simulink model "PubIfDecisionLM_MDL"  (R2020b)
settings: configuration reference "DspaceConfig" (kept outside this file)
PostLoadFcn:
  | if any(exist('dsrtsu_mdlpostloadfcn', 'file') ~= 0), dsrtsu_mdlpostloadfcn('Execute', bdroot); end
InitFcn:
  | , if any(exist('dsmpb_private', 'file') ~= 0), dsmpb_private('dsmpb_mdlclblib', 'Init', bdroot); end,
undefined symbols (not defined in the file or in its folder): OFM_OBJ_FUSIONTYPE_E, OFM_OBJ_MOVINGSTATE_E, OFM_OBJ_ORIENTATION_E, OFM_OBJ_TYPE_E, P_LM_Cyc, P_LM_EMLHistKapRcdBufSize, P_LM_EMLHistTrajBaseDis, P_LM_EMLHistTrajPNum, P_LM_EMLKapCorrMaxThre, P_LM_EMLMinKapThre, P_LM_EMLPathDisDiffThre, P_LM_EMLQuaFiltPar, P_LM_EMLTurnActKapThre, P_LM_EMLValidQuaThre, P_LM_FntPath1Disgap, P_LM_FntPath1MinDis, P_LM_FntPath1Timegap, P_LM_FntPath2Disgap, P_LM_FntPath2MinDis, P_LM_FntPath2Timegap, P_LM_FntPath3Disgap, P_LM_FntPath3MinDis, P_LM_FntPath3Timegap, P_LM_FusBLParFiltP, P_LM_FusEVDifC2Thre, P_LM_FusEVOPath1AllVSLDisThre, P_LM_FusEVOPath1AllVSLLostNumThre, P_LM_FusEVOPath1AllVSLQuaThre, P_LM_FusEVOPath1OTLFacNLC, P_LM_FusOTLQuaThre, P_LM_FusOTLSW, P_LM_FusParC0Index, P_LM_FusParC1Index, P_LM_FusParC2Index, P_LM_FusParC3Index, P_LM_FusVSLQuaThre, P_LM_FusVSLSW, P_LM_FusVSLValidSteerWheerAngThre, P_LM_FusVSLValidVxvThre, P_LM_LaneWidth, P_LM_OTLBufTPInfoEvaFactor, P_LM_OTLObjNum, P_LM_OTLObjSelectAgeThre, P_LM_OTLObjSelectDxAssessVx, P_LM_OTLObjSelectDxThre, P_LM_OTLObjSelectVxThre, P_LM_OTLObjSelectVyAssessDx, P_LM_OTLObjSelectVyThre, P_LM_OTLTrajPntBaseDis, P_LM_OTLTrajStdThre, P_LM_VSLAvailLineNum, P_LM_VSLBLSDiffThre, P_LM_VSLBLSDisRatio, P_LM_VSLFusBLParFiltP_C1, P_LM_VSLFusBLParFiltP_C2, P_LM_VSLFusBLParFiltP_C3, P_LM_VSLFusBLParFiltP_Quality, P_LM_VSLHistTrajBaseDis, P_LM_VSLHistTrajPNum, P_LM_VSLLCC0diff ... (+18)
libraries: simulink x145, LM_LIB x43
(part 5 of 24)

== system PubIfDecisionLM_MDL/Subsystem2/LM_OTL/LM_OTL_MovObjTrajRecord3/LM_OTL_BufTPCC ==
  LM_OTLBufTPVectBusK1 : Inport
  LM_VCAN_ESP : Inport  Port=2
  LM_ComBus : Inport  Port=3
  Bus Creator : BusCreator  Inputs=12
  Bus Selector : BusSelector  OutputSignals=LM_OTLBufL1DxVect,LM_OTLBufL1DyVect,LM_OTLBufL2DxVect,LM_OTLBufL2DyVect,LM_OTLBufE1DxVect,LM_OTLBufE1DyVect,LM_OTLBufE2DxVect,LM_OTLBufE2DyVect,LM_OTLBufR1DxVect,LM_OTLBufR1DyVect,LM_OTLBufR2DxVect,LM_OTLBufR2DyVect
  Bus Selector2 : BusSelector  OutputSignals=signal7.LM_ComEVOffsetX,signal7.LM_ComEVOffsetY,signal7.LM_ComEVOffsetAng
  Bus Selector5 : BusSelector  OutputSignals=VehStandstill
  Subsystem : Subsystem
  LM_OTLBufTPVectAdjuBus : Outport
  wires:
  LM_OTLBufTPVectBusK1/1 -> Bus Selector/1
  Subsystem/1(LM_OTLBufL1DxVectK1Adju) -> Bus Creator/1  "LM_OTLBufL1DxVectK1Adju"
  Bus Selector/11 -> Subsystem/15(LM_OTLBufR2DxVectK1)  "<LM_OTLBufR2DxVect>"
  Bus Selector/4 -> Subsystem/8(LM_OTLBufL2DyVectK1)  "<LM_OTLBufL2DyVect>"
  Bus Selector/5 -> Subsystem/9(LM_OTLBufE1DxVectK1)  "<LM_OTLBufE1DxVect>"
  Subsystem/5(LM_OTLBufE1DxVectK1Adju) -> Bus Creator/5  "LM_OTLBufE1DxVectK1Adju"
  Bus Selector/10 -> Subsystem/14(LM_OTLBufR1DyVectK1)  "<LM_OTLBufR1DyVect>"
  Bus Selector/8 -> Subsystem/12(LM_OTLBufE2DyVectK1)  "<LM_OTLBufE2DyVect>"
  Bus Selector/9 -> Subsystem/13(LM_OTLBufR1DxVectK1)  "<LM_OTLBufR1DxVect>"
  Bus Selector/7 -> Subsystem/11(LM_OTLBufE2DxVectK1)  "<LM_OTLBufE2DxVect>"
  Bus Selector/6 -> Subsystem/10(LM_OTLBufE1DyVectK1)  "<LM_OTLBufE1DyVect>"
  LM_VCAN_ESP/1 -> Bus Selector5/1
  Bus Selector/3 -> Subsystem/7(LM_OTLBufL2DxVectK1)  "<LM_OTLBufL2DxVect>"
  Subsystem/4(LM_OTLBufL2DyVectK1Adju) -> Bus Creator/4  "LM_OTLBufL2DyVectK1Adju"
  Bus Selector/2 -> Subsystem/6(LM_OTLBufL1DyVectK1)  "<LM_OTLBufL1DyVect>"
  Bus Selector/1 -> Subsystem/5(LM_OTLBufL1DxVectK1)  "<LM_OTLBufL1DxVect>"
  Subsystem/12(LM_OTLBufR2DyVectK1Adju) -> Bus Creator/12  "LM_OTLBufR2DyVectK1Adju"
  Subsystem/7(LM_OTLBufE2DxVectK1Adju) -> Bus Creator/7  "LM_OTLBufE2DxVectK1Adju"
  Subsystem/8(LM_OTLBufE2DyVectK1Adju) -> Bus Creator/8  "LM_OTLBufE2DyVectK1Adju"
  Subsystem/10(LM_OTLBufR1DyVectK1Adju) -> Bus Creator/10  "LM_OTLBufR1DyVectK1Adju"
  Bus Creator/1 -> LM_OTLBufTPVectAdjuBus/1  "LM_OTLBufTPVectAdjuBus"
  Bus Selector/12 -> Subsystem/16(LM_OTLBufR2DyVectK1)  "<LM_OTLBufR2DyVect>"
  Subsystem/9(LM_OTLBufR1DxVectK1Adju) -> Bus Creator/9  "LM_OTLBufR1DxVectK1Adju"
  Subsystem/6(LM_OTLBufE1DyVectK1Adju) -> Bus Creator/6  "LM_OTLBufE1DyVectK1Adju"
  Subsystem/11(LM_OTLBufR2DxVectK1Adju) -> Bus Creator/11  "LM_OTLBufR2DxVectK1Adju"
  Subsystem/2(LM_OTLBufL1DyVectK1Adju) -> Bus Creator/2  "LM_OTLBufL1DyVectK1Adju"
  Subsystem/3(LM_OTLBufL2DxVectK1Adju) -> Bus Creator/3  "LM_OTLBufL2DxVectK1Adju"
  Bus Selector2/1 -> Subsystem/2(LM_OTLOffsetX)  "<LM_ComEVOffsetX>"
  Bus Selector2/2 -> Subsystem/3(LM_OTLOffsetY)  "<LM_ComEVOffsetY>"
  Bus Selector2/3 -> Subsystem/4(LM_OTLOffsetAng)  "<LM_ComEVOffsetAng>"
  LM_ComBus/1 -> Bus Selector2/1
  Bus Selector5/1 -> Subsystem/1(VehStandstill)  "<VehStandstill>"

== system PubIfDecisionLM_MDL/Subsystem2/LM_OTL/LM_OTL_MovObjTrajRecord3/LM_OTL_MovObjSelc ==
  vxvRefMs : Inport
  OFM_OBJS : Inport  Port=2  OutDataTypeStr=Bus: OFM_OBJ_BUS
  Bus Creator : BusCreator  Inputs=6
  Bus Selector : BusSelector  OutputSignals=Object_DX,Object_DY
  Bus Selector1 : BusSelector  OutputSignals=Object_ID,Object_Type,Object_MovingState,Object_VX,Object_Orientation,Object_Fus_Type,Object_ExistProb,Object_VY,Object_DX,Object_Age
  Constant1 : Constant  Value=P_LM_OTLObjNum  OutDataTypeStr=uint8
  Data Type Conversion{,1..5} (6 alike) : DataTypeConversion  OutDataTypeStr=uint8
  LM_OTL_MovObjInterestedSelc : Subsystem
  Subsystem3 : Subsystem
  LM_OTLInterestObjIndexBus : Outport
  wires:
  vxvRefMs/1 -> Subsystem3/1(vxvRefMs)  "vxvRefMs"
  OFM_OBJS/1 -> Bus Selector/1, Bus Selector1/1
  Bus Selector1/10 -> Subsystem3/11(<Object_Age>)  "<Object_Age>"
  Bus Selector1/9 -> Subsystem3/10(<Object_DX>)  "<Object_DX>"
  Bus Selector1/8 -> Subsystem3/9(<Object_VY>)  "<Object_VY>"
  Bus Selector1/7 -> Subsystem3/8(<Object_ExistProb>)  "<Object_ExistProb>"
  Bus Selector1/6 -> Subsystem3/7(<Object_Fus_Type>)  "<Object_Fus_Type>"
  Bus Selector1/5 -> Subsystem3/6(<Object_Orientation>)  "<Object_Orientation>"
  Bus Selector1/4 -> Subsystem3/5(<Object_VX>)  "<Object_VX>"
  Bus Selector1/3 -> Subsystem3/4(<Object_MovingState>)  "<Object_MovingState>"
  Bus Selector1/2 -> Subsystem3/3(<Object_Type>)  "<Object_Type>"
  Bus Selector1/1 -> Subsystem3/2(<Object_ID>)  "<Object_ID>"
  Bus Selector/2 -> LM_OTL_MovObjInterestedSelc/4(Object_DY)  "<Object_DY>"
  Bus Selector/1 -> LM_OTL_MovObjInterestedSelc/3(Object_DX)  "<Object_DX>"
  Bus Creator/1 -> LM_OTLInterestObjIndexBus/1  "LM_OTLObjIndex"
  LM_OTL_MovObjInterestedSelc/6(LM_OTLRigObj2Index) -> Data Type Conversion5/1
  LM_OTL_MovObjInterestedSelc/5(LM_OTLRigObj1Index) -> Data Type Conversion4/1
  LM_OTL_MovObjInterestedSelc/4(LM_OTLHostObj2Index) -> Data Type Conversion3/1
  LM_OTL_MovObjInterestedSelc/3(LM_OTLHostObj1Index) -> Data Type Conversion2/1
  LM_OTL_MovObjInterestedSelc/2(LM_OTLLeObj2Index) -> Data Type Conversion1/1
  LM_OTL_MovObjInterestedSelc/1(LM_OTLLeObj1Index) -> Data Type Conversion/1
  Subsystem3/1(LM_OTL_MovObjValid) -> LM_OTL_MovObjInterestedSelc/1(LM_OTL_MovObjValid)  "LM_OTL_MovObjValid"
  Constant1/1 -> LM_OTL_MovObjInterestedSelc/2(P_LM_ObjNum)
  Data Type Conversion/1 -> Bus Creator/1  "LM_OTLCurLeLaObj1Index"
  Data Type Conversion1/1 -> Bus Creator/2  "LM_OTLCurLeLaObj2Index"
  Data Type Conversion2/1 -> Bus Creator/3  "LM_OTLCurEgoLaObj1Index"
  Data Type Conversion4/1 -> Bus Creator/5  "LM_OTLCurRigLaObj1Index"
  Data Type Conversion5/1 -> Bus Creator/6  "LM_OTLCurRigLaObj2Index"
  Data Type Conversion3/1 -> Bus Creator/4  "LM_OTLCurEgoLaObj2Index"

== system PubIfDecisionLM_MDL/Subsystem2/LM_OTL/LM_OTL_MovObjTrajRecord3/LM_OTL_ObjAlreadyRcdedJudge ==
  note: 判断当前周期感兴趣目标是否已经存储
  Object_ID : Inport  BusOutputAsStruct=on
  LM_OTLBufTPInfoBusK1 : Inport  Port=2
  LM_OTLInterestObjIndexBus : Inport  Port=3
  Bus Creator : BusCreator  Inputs=6
  Bus Creator1 : BusCreator  Inputs=6
  Bus Selector : BusSelector  OutputSignals=LM_OTLCurLeLaObj1Index,LM_OTLCurLeLaObj2Index,LM_OTLCurEgoLaObj1Index,LM_OTLCurEgoLaObj2Index,LM_OTLCurRigLaObj1Index,LM_OTLCurRigLaObj2Index
  Bus Selector1 : BusSelector  OutputSignals=LM_OTLCurLeLaObj1ID,LM_OTLCurLeLaObj2ID
  Bus Selector2 : BusSelector  OutputSignals=LM_OTLBufObjIDInfo.LM_OTLBufL1ObjID,LM_OTLBufObjIDInfo.LM_OTLBufL2ObjID
  Bus Selector3 : BusSelector  OutputSignals=LM_OTLCurEgoLaObj1ID,LM_OTLCurEgoLaObj2ID
  Bus Selector4 : BusSelector  OutputSignals=LM_OTLCurRigLaObj1ID,LM_OTLCurRigLaObj2ID
  Bus Selector5 : BusSelector  OutputSignals=LM_OTLBufObjIDInfo.LM_OTLBufE1ObjID,LM_OTLBufObjIDInfo.LM_OTLBufE2ObjID
  Bus Selector6 : BusSelector  OutputSignals=LM_OTLBufObjIDInfo.LM_OTLBufR1ObjID,LM_OTLBufObjIDInfo.LM_OTLBufR2ObjID
  LM_OTL_CurObjIDCalc : Subsystem
  LM_OTL_EglLaneRcdJudge : Subsystem
  LM_OTL_LeLaneRcdJudge : Subsystem
  LM_OTL_RigLaneRcdJudge : Subsystem
  LM_OTLCurObjIDBus : Outport
  LM_OTLObjRcdedFlg_Bus : Outport  Port=2
  wires:
  LM_OTLInterestObjIndexBus/1 -> Bus Selector/1
  LM_OTL_LeLaneRcdJudge/1(LM_OTLCurLeLaObj1RcdedFlg) -> Bus Creator/1
  LM_OTL_LeLaneRcdJudge/2(LM_OTLCurLeLaObj2RcdedFlg) -> Bus Creator/2
  LM_OTL_EglLaneRcdJudge/1(LM_OTLCurEgoLaObj1RcdedFlg) -> Bus Creator/3
  LM_OTL_EglLaneRcdJudge/2(LM_OTLCurEgoLaObj2RcdedFlg) -> Bus Creator/4
  LM_OTL_RigLaneRcdJudge/1(LM_OTLCurRigLaObj1RcdedFlg) -> Bus Creator/5
  LM_OTL_RigLaneRcdJudge/2(LM_OTLCurRigLaObj2RcdedFlg) -> Bus Creator/6
  Bus Creator/1 -> LM_OTLObjRcdedFlg_Bus/1  "LM_OTLObjRcdedFlg_Bus"
  Object_ID/1 -> LM_OTL_CurObjIDCalc/1(Object_ID)
  Bus Selector/1 -> LM_OTL_CurObjIDCalc/2(LM_OTLCurLeLaObj1Index)  "<LM_OTLCurLeLaObj1Index>"
  Bus Selector/2 -> LM_OTL_CurObjIDCalc/3(LM_OTLCurLeLaObj2Index)  "<LM_OTLCurLeLaObj2Index>"
  Bus Selector/3 -> LM_OTL_CurObjIDCalc/4(LM_OTLCurEgoLaObj1Index)  "<LM_OTLCurEgoLaObj1Index>"
  Bus Selector/4 -> LM_OTL_CurObjIDCalc/5(LM_OTLCurEgoLaObj2Index)  "<LM_OTLCurEgoLaObj2Index>"
  Bus Selector/5 -> LM_OTL_CurObjIDCalc/6(LM_OTLCurRigLaObj1Index)  "<LM_OTLCurRigLaObj1Index>"
  Bus Selector/6 -> LM_OTL_CurObjIDCalc/7(LM_OTLCurRigLaObj2Index)  "<LM_OTLCurRigLaObj2Index>"
  LM_OTL_CurObjIDCalc/1(LM_OTLCurLeLaObj1ID) -> Bus Creator1/1
  LM_OTL_CurObjIDCalc/2(LM_OTLCurLeLaObj2ID) -> Bus Creator1/2
  LM_OTL_CurObjIDCalc/3(LM_OTLCurEgoLaObj1ID) -> Bus Creator1/3
  LM_OTL_CurObjIDCalc/4(LM_OTLCurEgoLaObj2ID) -> Bus Creator1/4
  LM_OTL_CurObjIDCalc/5(LM_OTLCurRigLaObj1ID) -> Bus Creator1/5
  LM_OTL_CurObjIDCalc/6(LM_OTLCurRigLaObj2ID) -> Bus Creator1/6
  Bus Selector1/1 -> LM_OTL_LeLaneRcdJudge/1(LM_OTLCurLeLa1ObjID)  "<LM_OTLCurLeLaObj1ID>"
  Bus Selector1/2 -> LM_OTL_LeLaneRcdJudge/2(LM_OTLCurLeLa2ObjID)  "<LM_OTLCurLeLaObj2ID>"
  Bus Creator1/1 -> LM_OTLCurObjIDBus/1, Bus Selector4/1, Bus Selector3/1, Bus Selector1/1
  LM_OTLBufTPInfoBusK1/1 -> Bus Selector6/1, Bus Selector5/1, Bus Selector2/1
  Bus Selector2/1 -> LM_OTL_LeLaneRcdJudge/3(LM_OTLBufL1ObjIDK1)  "<LM_OTLBufL1ObjID>"
  Bus Selector2/2 -> LM_OTL_LeLaneRcdJudge/4(LM_OTLBufL2ObjIDK1)  "<LM_OTLBufL2ObjID>"
  Bus Selector3/1 -> LM_OTL_EglLaneRcdJudge/1(LM_OTLCurEgoLa1ObjID)  "<LM_OTLCurEgoLaObj1ID>"
  Bus Selector3/2 -> LM_OTL_EglLaneRcdJudge/2(LM_OTLCurEgoLa2ObjID)  "<LM_OTLCurEgoLaObj2ID>"
  Bus Selector4/1 -> LM_OTL_RigLaneRcdJudge/1(LM_OTLCurRigLa1ObjID)  "<LM_OTLCurRigLaObj1ID>"
  Bus Selector4/2 -> LM_OTL_RigLaneRcdJudge/2(LM_OTLCurRigLa2ObjID)  "<LM_OTLCurRigLaObj2ID>"
  Bus Selector5/1 -> LM_OTL_EglLaneRcdJudge/3(LM_OTLBufE1ObjIDK1)  "<LM_OTLBufE1ObjID>"
  Bus Selector5/2 -> LM_OTL_EglLaneRcdJudge/4(LM_OTLBufE2ObjIDK1)  "<LM_OTLBufE2ObjID>"
  Bus Selector6/1 -> LM_OTL_RigLaneRcdJudge/3(LM_OTLBufR1ObjIDK1)  "<LM_OTLBufR1ObjID>"
  Bus Selector6/2 -> LM_OTL_RigLaneRcdJudge/4(LM_OTLBufR2ObjIDK1)  "<LM_OTLBufR2ObjID>"

== system PubIfDecisionLM_MDL/Subsystem2/LM_OTL/LM_OTL_MovObjTrajRecord3/LM_OTL_ObjRcdFlgJudge ==
  LM_OTLObjRcdedFlg_Bus : Inport
  Object_Dx : Inport  Port=2
  Object_Dy : Inport  Port=3
  LM_OTLInterestObjIndexBus : Inport  Port=4
  LM_OTLBufTPVectAdjuBus : Inport  Port=5
  LM_OTLBufTPInfoBusK1 : Inport  Port=6
  Bus Creator : BusCreator  Inputs=12
  Bus Creator1 : BusCreator  Inputs=6
  Bus Creator2 : BusCreator  Inputs=6
  Bus Selector : BusSelector  OutputSignals=LM_OTLCurLeLaObj1RcdedFlg,LM_OTLCurLeLaObj2RcdedFlg
  Bus Selector1 : BusSelector  OutputSignals=LM_OTLCurEgoLaObj1RcdedFlg,LM_OTLCurEgoLaObj2RcdedFlg
  Bus Selector10 : BusSelector  OutputSignals=LM_OTLBufLe1ObjDxK1,LM_OTLBufLe2ObjDxK1
  Bus Selector11 : BusSelector  OutputSignals=LM_OTLBufEgo1ObjDxK1,LM_OTLBufEgo2ObjDxK1
  Bus Selector12 : BusSelector  OutputSignals=LM_OTLBufRig1ObjDxK1,LM_OTLBufRig2ObjDxK1
  Bus Selector13 : BusSelector  OutputSignals=LM_OTLBufL1DxVectK1Adju,LM_OTLBufL2DxVectK1Adju,LM_OTLBufE1DxVectK1Adju,LM_OTLBufE2DxVectK1Adju,LM_OTLBufR1DxVectK1Adju,LM_OTLBufR2DxVectK1Adju
  Bus Selector14 : BusSelector  OutputSignals=LM_OTLBufEPPosInfo.LM_OTLBufL1EPPos,LM_OTLBufEPPosInfo.LM_OTLBufL2EPPos,LM_OTLBufEPPosInfo.LM_OTLBufE1EPPos,LM_OTLBufEPPosInfo.LM_OTLBufE2EPPos,LM_OTLBufEPPosInfo.LM_OTLBufR1EPPos,LM_OTLBufEPPosInfo.LM_OTLBufR2EPPos
  Bus Selector2 : BusSelector  OutputSignals=LM_OTLCurLeLaObj1Index,LM_OTLCurLeLaObj2Index,LM_OTLCurEgoLaObj1Index,LM_OTLCurEgoLaObj2Index,LM_OTLCurRigLaObj1Index,LM_OTLCurRigLaObj2Index
  Bus Selector3 : BusSelector  OutputSignals=LM_OTLCurRigLaObj1RcdedFlg,LM_OTLCurRigLaObj2RcdedFlg
  Bus Selector4 : BusSelector  OutputSignals=LM_OTLCurLeLaObj1Index,LM_OTLCurLeLaObj2Index
  Bus Selector5 : BusSelector  OutputSignals=LM_OTLCurEgoLaObj1Index,LM_OTLCurEgoLaObj2Index
  Bus Selector6 : BusSelector  OutputSignals=LM_OTLCurRigLaObj1Index,LM_OTLCurRigLaObj2Index
  Bus Selector7 : BusSelector  OutputSignals=LM_OTLCurLeLaObj1Dx,LM_OTLCurLeLaObj2Dx
  Bus Selector8 : BusSelector  OutputSignals=LM_OTLCurEgoLaObj1Dx,LM_OTLCurEgoLaObj2Dx
  Bus Selector9 : BusSelector  OutputSignals=LM_OTLCurRigLaObj1Dx,LM_OTLCurRigLaObj2Dx
  LM_OTL_BufObjEndDxCalc : Subsystem
  LM_OTL_CurObjDxCalc : Subsystem
  LM_OTL_EgoLaObjRcdFlgJudge : Subsystem
  LM_OTL_LeLaObjRcdFlgJudge : Subsystem
  LM_OTL_RigLaObjRcdFlgJudge : Subsystem
  LM_OTLCurObjRcdFlgBus : Outport
  LM_OTLCurObjPositonBus : Outport  Port=2
  wires:
  Bus Selector14/6 -> LM_OTL_BufObjEndDxCalc/12(LM_OTLBufRig2ObjPEndIndexK1)  "<LM_OTLBufR2EPPos>"
  Bus Selector14/5 -> LM_OTL_BufObjEndDxCalc/11(LM_OTLBufRig1ObjPEndIndexK1)  "<LM_OTLBufR1EPPos>"
  Bus Selector14/4 -> LM_OTL_BufObjEndDxCalc/10(LM_OTLBufEgo2ObjPEndIndexK1)  "<LM_OTLBufE2EPPos>"
  Bus Selector14/3 -> LM_OTL_BufObjEndDxCalc/9(LM_OTLBufEgo1ObjPEndIndexK1)  "<LM_OTLBufE1EPPos>"
  Bus Selector14/2 -> LM_OTL_BufObjEndDxCalc/8(LM_OTLBufLe2ObjPEndIndexK1)  "<LM_OTLBufL2EPPos>"
  Bus Selector14/1 -> LM_OTL_BufObjEndDxCalc/7(LM_OTLBufLe1ObjPEndIndexK1)  "<LM_OTLBufL1EPPos>"
  Bus Selector13/6 -> LM_OTL_BufObjEndDxCalc/6(LM_OTLBufRig2ObjDxVectK1)  "<LM_OTLBufR2DxVectK1Adju>"
  Bus Selector13/5 -> LM_OTL_BufObjEndDxCalc/5(LM_OTLBufRig1ObjDxVectK1)  "<LM_OTLBufR1DxVectK1Adju>"
  Bus Selector13/4 -> LM_OTL_BufObjEndDxCalc/4(LM_OTLBufEgo2ObjDxVectK1)  "<LM_OTLBufE2DxVectK1Adju>"
  Bus Selector13/3 -> LM_OTL_BufObjEndDxCalc/3(LM_OTLBufEgo1ObjDxVectK1)  "<LM_OTLBufE1DxVectK1Adju>"
  Bus Selector13/2 -> LM_OTL_BufObjEndDxCalc/2(LM_OTLBufLe2ObjDxVectK1)  "<LM_OTLBufL2DxVectK1Adju>"
  Bus Selector13/1 -> LM_OTL_BufObjEndDxCalc/1(LM_OTLBufLe1ObjDxVectK1)  "<LM_OTLBufL1DxVectK1Adju>"
  LM_OTLBufTPInfoBusK1/1 -> Bus Selector14/1
  LM_OTLBufTPVectAdjuBus/1 -> Bus Selector13/1
  LM_OTLObjRcdedFlg_Bus/1 -> Bus Selector/1, Bus Selector3/1, Bus Selector1/1
  Bus Selector/1 -> LM_OTL_LeLaObjRcdFlgJudge/1(LM_OTLCurLeLaObj1RcdedFlg)  "<LM_OTLCurLeLaObj1RcdedFlg>"
  Bus Selector/2 -> LM_OTL_LeLaObjRcdFlgJudge/2(LM_OTLCurLeLaObj2RcdedFlg)  "<LM_OTLCurLeLaObj2RcdedFlg>"
  LM_OTLInterestObjIndexBus/1 -> [LM_OTLInterestObjIndexBus], Bus Selector2/1
  Bus Selector2/1 -> LM_OTL_CurObjDxCalc/3(LM_OTLCurLeLaObj1Index)  "<LM_OTLCurLeLaObj1Index>"
  Bus Selector2/2 -> LM_OTL_CurObjDxCalc/4(LM_OTLCurLeLaObj2Index)  "<LM_OTLCurLeLaObj2Index>"
  Bus Selector2/3 -> LM_OTL_CurObjDxCalc/5(LM_OTLCurEgoLaObj1Index)  "<LM_OTLCurEgoLaObj1Index>"
  Bus Selector2/4 -> LM_OTL_CurObjDxCalc/6(LM_OTLCurEgoLaObj2Index)  "<LM_OTLCurEgoLaObj2Index>"
  Bus Selector2/5 -> LM_OTL_CurObjDxCalc/7(LM_OTLCurRigLaObj1Index)  "<LM_OTLCurRigLaObj1Index>"
  Bus Selector2/6 -> LM_OTL_CurObjDxCalc/8(LM_OTLCurRigLaObj2Index)  "<LM_OTLCurRigLaObj2Index>"
  Bus Creator/1 -> LM_OTLCurObjPositonBus/1, Bus Selector7/1, Bus Selector8/1, Bus Selector9/1  "LM_OTLCurObjDxBus"
  Bus Selector1/1 -> LM_OTL_EgoLaObjRcdFlgJudge/1(LM_OTLCurEgoLaObj1RcdedFlg)  "<LM_OTLCurEgoLaObj1RcdedFlg>"
  Bus Selector1/2 -> LM_OTL_EgoLaObjRcdFlgJudge/2(LM_OTLCurEgoLaObj2RcdedFlg)  "<LM_OTLCurEgoLaObj2RcdedFlg>"
  Bus Selector3/1 -> LM_OTL_RigLaObjRcdFlgJudge/7(LM_OTLCurRigLaObj1RcdedFlg)  "<LM_OTLCurRigLaObj1RcdedFlg>"
  Bus Selector3/2 -> LM_OTL_RigLaObjRcdFlgJudge/8(LM_OTLCurRigLaObj2RcdedFlg)  "<LM_OTLCurRigLaObj2RcdedFlg>"
  Object_Dx/1 -> LM_OTL_CurObjDxCalc/1(Object_Dx)
  Bus Selector4/2 -> LM_OTL_LeLaObjRcdFlgJudge/4(LM_OTLCurLeLaObj2Index)  "<LM_OTLCurLeLaObj2Index>"
  Bus Selector4/1 -> LM_OTL_LeLaObjRcdFlgJudge/3(LM_OTLCurLeLaObj1Index)  "<LM_OTLCurLeLaObj1Index>"
  [LM_OTLInterestObjIndexBus] -> Bus Selector5/1, Bus Selector6/1, Bus Selector4/1
  Bus Selector5/1 -> LM_OTL_EgoLaObjRcdFlgJudge/3(LM_OTLCurEgoLaObj1Index)  "<LM_OTLCurEgoLaObj1Index>"
  Bus Selector5/2 -> LM_OTL_EgoLaObjRcdFlgJudge/4(LM_OTLCurEgoLaObj2Index)  "<LM_OTLCurEgoLaObj2Index>"
  Bus Selector6/1 -> LM_OTL_RigLaObjRcdFlgJudge/1(LM_OTLCurRigLaObj1Index)  "<LM_OTLCurRigLaObj1Index>"
  Bus Selector6/2 -> LM_OTL_RigLaObjRcdFlgJudge/2(LM_OTLCurRigLaObj2Index)  "<LM_OTLCurRigLaObj2Index>"
  Bus Selector7/1 -> LM_OTL_LeLaObjRcdFlgJudge/5(LM_OTLCurLeLaObj1Dx)  "<LM_OTLCurLeLaObj1Dx>"
  Bus Selector7/2 -> LM_OTL_LeLaObjRcdFlgJudge/6(LM_OTLCurLeLaObj2Dx)  "<LM_OTLCurLeLaObj2Dx>"
  Bus Selector8/1 -> LM_OTL_EgoLaObjRcdFlgJudge/5(LM_OTLCurEgoLaObj1Dx)  "<LM_OTLCurEgoLaObj1Dx>"
  Bus Selector8/2 -> LM_OTL_EgoLaObjRcdFlgJudge/6(LM_OTLCurEgoLaObj2Dx)  "<LM_OTLCurEgoLaObj2Dx>"
  Bus Selector9/1 -> LM_OTL_RigLaObjRcdFlgJudge/3(LM_OTLCurRigLaObj1Dx)  "<LM_OTLCurRigLaObj1Dx>"
  Bus Selector9/2 -> LM_OTL_RigLaObjRcdFlgJudge/4(LM_OTLCurRigLaObj2Dx)  "<LM_OTLCurRigLaObj2Dx>"
  LM_OTL_BufObjEndDxCalc/1(LM_OTLBufLe1ObjDxK1) -> Bus Creator1/1
  LM_OTL_BufObjEndDxCalc/2(LM_OTLBufLe2ObjDxK1) -> Bus Creator1/2
  LM_OTL_BufObjEndDxCalc/3(LM_OTLBufEgo1ObjDxK1) -> Bus Creator1/3
  LM_OTL_BufObjEndDxCalc/4(LM_OTLBufEgo2ObjDxK1) -> Bus Creator1/4
  LM_OTL_BufObjEndDxCalc/5(LM_OTLBufRig1ObjDxK1) -> Bus Creator1/5
  LM_OTL_BufObjEndDxCalc/6(LM_OTLBufRig2ObjDxK1) -> Bus Creator1/6
  Bus Selector10/1 -> LM_OTL_LeLaObjRcdFlgJudge/7(LM_OTLBufLe1ObjDxK1)  "<LM_OTLBufLe1ObjDxK1>"
  Bus Creator1/1 -> Bus Selector12/1, Bus Selector10/1, Bus Selector11/1
  Bus Selector10/2 -> LM_OTL_LeLaObjRcdFlgJudge/8(LM_OTLBufLe2ObjDxK1)  "<LM_OTLBufLe2ObjDxK1>"
  Bus Selector11/1 -> LM_OTL_EgoLaObjRcdFlgJudge/7(LM_OTLBufEgo1ObjDxK1)  "<LM_OTLBufEgo1ObjDxK1>"
  Bus Selector11/2 -> LM_OTL_EgoLaObjRcdFlgJudge/8(LM_OTLBufEgo2ObjDxK1)  "<LM_OTLBufEgo2ObjDxK1>"
  Bus Selector12/1 -> LM_OTL_RigLaObjRcdFlgJudge/5(LM_OTLBufRig1ObjDxK1)  "<LM_OTLBufRig1ObjDxK1>"
  Bus Selector12/2 -> LM_OTL_RigLaObjRcdFlgJudge/6(LM_OTLBufRig2ObjDxK1)  "<LM_OTLBufRig2ObjDxK1>"
  LM_OTL_LeLaObjRcdFlgJudge/1(LM_OTLCurLeLaObj1RcdFlg) -> Bus Creator2/1
  LM_OTL_LeLaObjRcdFlgJudge/2(LM_OTLCurLeLaObj2RcdFlg) -> Bus Creator2/2
  LM_OTL_EgoLaObjRcdFlgJudge/2(LM_OTLCurEgoLaObj2RcdFlg) -> Bus Creator2/4
  LM_OTL_EgoLaObjRcdFlgJudge/1(LM_OTLCurEgoLaObj1RcdFlg) -> Bus Creator2/3
  LM_OTL_RigLaObjRcdFlgJudge/1(LM_OTLCurRigLaObj1RcdFlg) -> Bus Creator2/5
  LM_OTL_RigLaObjRcdFlgJudge/2(LM_OTLCurRigLaObj2RcdFlg) -> Bus Creator2/6
  Bus Creator2/1 -> LM_OTLCurObjRcdFlgBus/1  "LM_OTLCurObjRcdFlgBus"
  Object_Dy/1 -> LM_OTL_CurObjDxCalc/2(Object_Dy)
  LM_OTL_CurObjDxCalc/2(LM_OTLCurLeLaObj1Dy) -> Bus Creator/2
  LM_OTL_CurObjDxCalc/1(LM_OTLCurLeLaObj1Dx) -> Bus Creator/1
  LM_OTL_CurObjDxCalc/3(LM_OTLCurLeLaObj2Dx) -> Bus Creator/3
  LM_OTL_CurObjDxCalc/4(LM_OTLCurLeLaObj2Dy) -> Bus Creator/4
  LM_OTL_CurObjDxCalc/5(LM_OTLCurEgoLaObj1Dx) -> Bus Creator/5
  LM_OTL_CurObjDxCalc/6(LM_OTLCurEgoLaObj1Dy) -> Bus Creator/6
  LM_OTL_CurObjDxCalc/7(LM_OTLCurEgoLaObj2Dx) -> Bus Creator/7
  LM_OTL_CurObjDxCalc/8(LM_OTLCurEgoLaObj2Dy) -> Bus Creator/8
  LM_OTL_CurObjDxCalc/9(LM_OTLCurRigLaObj1Dx) -> Bus Creator/9
  LM_OTL_CurObjDxCalc/10(LM_OTLCurRigLaObj1Dy) -> Bus Creator/10
  LM_OTL_CurObjDxCalc/11(LM_OTLCurRigLaObj2Dx) -> Bus Creator/11
  LM_OTL_CurObjDxCalc/12(LM_OTLCurRigLaObj2Dy) -> Bus Creator/12

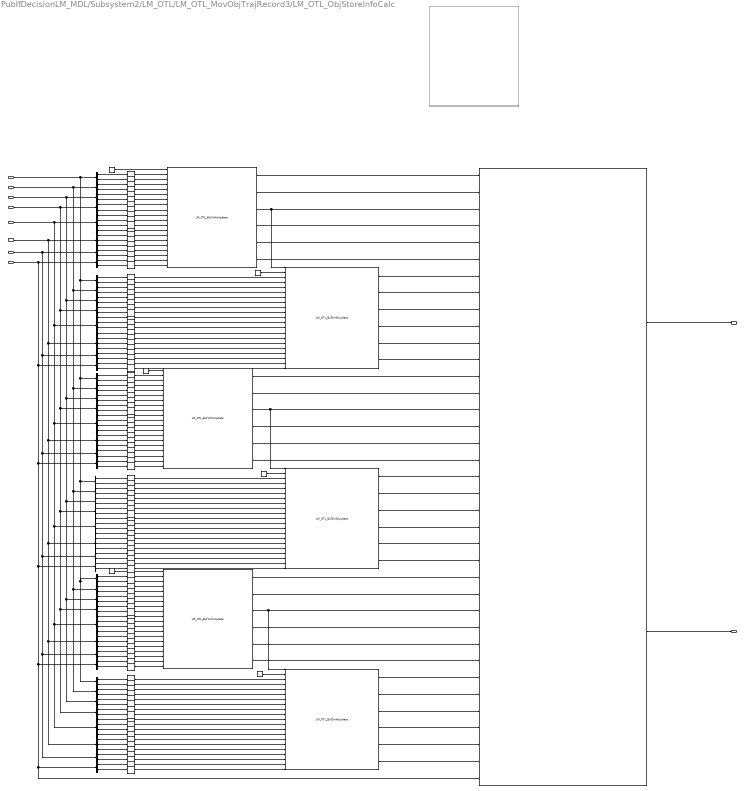
== system PubIfDecisionLM_MDL/Subsystem2/LM_OTL/LM_OTL_MovObjTrajRecord3/LM_OTL_ObjStoreInfoCalc ==
  LM_OTLBufTPVectAdjuBus : Inport
  LM_OTLCurObjIDBus : Inport  Port=2  BusOutputAsStruct=on
  LM_OTLObjRcdedFlg_Bus : Inport  Port=3  BusOutputAsStruct=on
  LM_OTLCurObjRcdFlgBus : Inport  Port=4
  LM_OTLCurObjPositonBus : Inport  Port=5  BusOutputAsStruct=on
  LM_OTLInterestObjIndexBus : Inport  Port=6
  LM_OTLBufTPInfoBusK1 : Inport  Port=7
  LM_OTLBufLastTPInfoBus : Inport  Port=8
  Bus Selector : BusSelector  OutputSignals=LM_OTLCurLeLaObj1RcdedFlg,LM_OTLCurLeLaObj2RcdedFlg
  Bus Selector1 : BusSelector  OutputSignals=LM_OTLCurLeLaObj1RcdFlg,LM_OTLCurLeLaObj2RcdFlg
  Bus Selector10 : BusSelector  OutputSignals=LM_OTLCurLeLaObj1ID,LM_OTLCurLeLaObj2ID
  Bus Selector11 : BusSelector  OutputSignals=LM_OTLCurLeLaObj1Dx,LM_OTLCurLeLaObj2Dx,LM_OTLCurLeLaObj1Dy,LM_OTLCurLeLaObj2Dy
  Bus Selector12 : BusSelector  OutputSignals=LM_OTLBufPNumInfo.LM_OTLBufL2PNum,LM_OTLBufSPPosInfo.LM_OTLBufL2SPPos,LM_OTLBufEPPosInfo.LM_OTLBufL2EPPos
  Bus Selector13 : BusSelector  OutputSignals=LM_OTLCurLeLaObj1Index,LM_OTLCurLeLaObj2Index
  Bus Selector14 : BusSelector  OutputSignals=LM_OTLBufL2LastTPInfo.LM_OTLBufL2LastTPValid,LM_OTLBufL2LastTPInfo.LM_OTLBufL2LastEPPos
  Bus Selector15 : BusSelector  OutputSignals=LM_OTLBufL2DxVectK1Adju,LM_OTLBufL2DyVectK1Adju
  Bus Selector16 : BusSelector  OutputSignals=LM_OTLCurEgoLaObj1ID,LM_OTLCurEgoLaObj2ID
  Bus Selector17 : BusSelector  OutputSignals=LM_OTLCurEgoLaObj1Dx,LM_OTLCurEgoLaObj2Dx,LM_OTLCurEgoLaObj1Dy,LM_OTLCurEgoLaObj2Dy
  Bus Selector18 : BusSelector  OutputSignals=LM_OTLBufPNumInfo.LM_OTLBufE1PNum,LM_OTLBufSPPosInfo.LM_OTLBufE1SPPos,LM_OTLBufEPPosInfo.LM_OTLBufE1EPPos
  Bus Selector19 : BusSelector  OutputSignals=LM_OTLCurEgoLaObj1Index,LM_OTLCurEgoLaObj2Index
  Bus Selector2 : BusSelector  OutputSignals=LM_OTLCurLeLaObj1ID,LM_OTLCurLeLaObj2ID
  Bus Selector20 : BusSelector  OutputSignals=LM_OTLBufE1LastTPInfo.LM_OTLBufE1LastTPValid,LM_OTLBufE1LastTPInfo.LM_OTLBufE1LastEPPos
  Bus Selector21 : BusSelector  OutputSignals=LM_OTLBufE1DxVectK1Adju,LM_OTLBufE1DyVectK1Adju
  Bus Selector22 : BusSelector  OutputSignals=LM_OTLCurEgoLaObj1RcdedFlg,LM_OTLCurEgoLaObj2RcdedFlg
  Bus Selector23 : BusSelector  OutputSignals=LM_OTLCurEgoLaObj1RcdFlg,LM_OTLCurEgoLaObj2RcdFlg
  Bus Selector24 : BusSelector  OutputSignals=LM_OTLCurEgoLaObj1ID,LM_OTLCurEgoLaObj2ID
  Bus Selector25 : BusSelector  OutputSignals=LM_OTLCurEgoLaObj1Dx,LM_OTLCurEgoLaObj2Dx,LM_OTLCurEgoLaObj1Dy,LM_OTLCurEgoLaObj2Dy
  Bus Selector26 : BusSelector  OutputSignals=LM_OTLBufPNumInfo.LM_OTLBufE2PNum,LM_OTLBufSPPosInfo.LM_OTLBufE2SPPos,LM_OTLBufEPPosInfo.LM_OTLBufE2EPPos
  Bus Selector27 : BusSelector  OutputSignals=LM_OTLCurEgoLaObj1Index,LM_OTLCurEgoLaObj2Index
  Bus Selector28 : BusSelector  OutputSignals=LM_OTLBufE2LastTPInfo.LM_OTLBufE2LastTPValid,LM_OTLBufE2LastTPInfo.LM_OTLBufE2LastEPPos
  Bus Selector29 : BusSelector  OutputSignals=LM_OTLBufE2DxVectK1Adju,LM_OTLBufE2DyVectK1Adju
  Bus Selector3 : BusSelector  OutputSignals=LM_OTLCurLeLaObj1Dx,LM_OTLCurLeLaObj2Dx,LM_OTLCurLeLaObj1Dy,LM_OTLCurLeLaObj2Dy
  Bus Selector30 : BusSelector  OutputSignals=LM_OTLCurEgoLaObj1RcdedFlg,LM_OTLCurEgoLaObj2RcdedFlg
  Bus Selector31 : BusSelector  OutputSignals=LM_OTLCurEgoLaObj1RcdFlg,LM_OTLCurEgoLaObj2RcdFlg
  Bus Selector32 : BusSelector  OutputSignals=LM_OTLCurRigLaObj1ID,LM_OTLCurRigLaObj2ID
  Bus Selector33 : BusSelector  OutputSignals=LM_OTLCurRigLaObj1Dx,LM_OTLCurRigLaObj2Dx,LM_OTLCurRigLaObj1Dy,LM_OTLCurRigLaObj2Dy
  Bus Selector34 : BusSelector  OutputSignals=LM_OTLBufPNumInfo.LM_OTLBufR1PNum,LM_OTLBufSPPosInfo.LM_OTLBufR1SPPos,LM_OTLBufEPPosInfo.LM_OTLBufR1EPPos
  Bus Selector35 : BusSelector  OutputSignals=LM_OTLCurRigLaObj1Index,LM_OTLCurRigLaObj2Index
  Bus Selector36 : BusSelector  OutputSignals=LM_OTLBufR1LastTPInfo.LM_OTLBufR1LastTPValid,LM_OTLBufR1LastTPInfo.LM_OTLBufR1LastEPPos
  Bus Selector37 : BusSelector  OutputSignals=LM_OTLBufR1DxVectK1Adju,LM_OTLBufR1DyVectK1Adju
  Bus Selector38 : BusSelector  OutputSignals=LM_OTLCurRigLaObj1RcdedFlg,LM_OTLCurRigLaObj2RcdedFlg
  Bus Selector39 : BusSelector  OutputSignals=LM_OTLCurRigLaObj1RcdFlg,LM_OTLCurRigLaObj2RcdFlg
  Bus Selector4 : BusSelector  OutputSignals=LM_OTLBufPNumInfo.LM_OTLBufL1PNum,LM_OTLBufSPPosInfo.LM_OTLBufL1SPPos,LM_OTLBufEPPosInfo.LM_OTLBufL1EPPos
  Bus Selector40 : BusSelector  OutputSignals=LM_OTLCurRigLaObj1ID,LM_OTLCurRigLaObj2ID
  Bus Selector41 : BusSelector  OutputSignals=LM_OTLCurRigLaObj1Dx,LM_OTLCurRigLaObj2Dx,LM_OTLCurRigLaObj1Dy,LM_OTLCurRigLaObj2Dy
  Bus Selector42 : BusSelector  OutputSignals=LM_OTLBufPNumInfo.LM_OTLBufR2PNum,LM_OTLBufSPPosInfo.LM_OTLBufR2SPPos,LM_OTLBufEPPosInfo.LM_OTLBufR2EPPos
  Bus Selector43 : BusSelector  OutputSignals=LM_OTLCurRigLaObj1Index,LM_OTLCurRigLaObj2Index
  Bus Selector44 : BusSelector  OutputSignals=LM_OTLBufR2LastTPInfo.LM_OTLBufR2LastTPValid,LM_OTLBufR2LastTPInfo.LM_OTLBufR2LastEPPos
  Bus Selector45 : BusSelector  OutputSignals=LM_OTLBufR2DxVectK1Adju,LM_OTLBufR2DyVectK1Adju
  Bus Selector46 : BusSelector  OutputSignals=LM_OTLCurRigLaObj1RcdedFlg,LM_OTLCurRigLaObj2RcdedFlg
  Bus Selector47 : BusSelector  OutputSignals=LM_OTLCurRigLaObj1RcdFlg,LM_OTLCurRigLaObj2RcdFlg
  Bus Selector5 : BusSelector  OutputSignals=LM_OTLCurLeLaObj1Index,LM_OTLCurLeLaObj2Index
  Bus Selector6 : BusSelector  OutputSignals=LM_OTLBufL1LastTPInfo.LM_OTLBufL1LastTPValid,LM_OTLBufL1LastTPInfo.LM_OTLBufL1LastEPPos
  Bus Selector7 : BusSelector  OutputSignals=LM_OTLBufL1DxVectK1Adju,LM_OTLBufL1DyVectK1Adju
  Bus Selector8 : BusSelector  OutputSignals=LM_OTLCurLeLaObj1RcdedFlg,LM_OTLCurLeLaObj2RcdedFlg
  Bus Selector9 : BusSelector  OutputSignals=LM_OTLCurLeLaObj1RcdFlg,LM_OTLCurLeLaObj2RcdFlg
  Constant : Constant  OutDataTypeStr=uint8
  Constant1 : Constant  Value=2  OutDataTypeStr=uint8
  Constant2 : Constant  OutDataTypeStr=uint8
  Constant3 : Constant  Value=2  OutDataTypeStr=uint8
  Constant4 : Constant  OutDataTypeStr=uint8
  Constant5 : Constant  Value=2  OutDataTypeStr=uint8
  LM_OTL_Buf1InfoUpdate : LM_LIB/LM_OTL_Buf1InfoUpdate  SystemSampleTime=-1  VariantActivationTime=update diagram  Latency=0  AutoFrameSizeCalculation=off
  LM_OTL_Buf1InfoUpdate1 : LM_LIB/LM_OTL_Buf1InfoUpdate  SystemSampleTime=-1  VariantActivationTime=update diagram  Latency=0  AutoFrameSizeCalculation=off
  LM_OTL_Buf1InfoUpdate2 : LM_LIB/LM_OTL_Buf1InfoUpdate  SystemSampleTime=-1  VariantActivationTime=update diagram  Latency=0  AutoFrameSizeCalculation=off
  LM_OTL_Buf2InfoUpdate : LM_LIB/LM_OTL_Buf2InfoUpdate  SystemSampleTime=-1  VariantActivationTime=update diagram  Latency=0  AutoFrameSizeCalculation=off
  LM_OTL_Buf2InfoUpdate1 : LM_LIB/LM_OTL_Buf2InfoUpdate  SystemSampleTime=-1  VariantActivationTime=update diagram  Latency=0  AutoFrameSizeCalculation=off
  LM_OTL_Buf2InfoUpdate2 : LM_LIB/LM_OTL_Buf2InfoUpdate  SystemSampleTime=-1  VariantActivationTime=update diagram  Latency=0  AutoFrameSizeCalculation=off
  LM_OTL_BufLe1InfoUpdate1 : Subsystem  Commented=on
  Signal Conversion{2..115} (114 alike) : SignalConversion  OverrideOpt=off
  Subsystem : Subsystem
  LM_OTLBufTPVectBus : Outport
  LM_OTLBufTPInfoBus : Outport  Port=2
  wires:
  Signal Conversion97/1 -> LM_OTL_Buf1InfoUpdate/10
  Signal Conversion107/1 -> LM_OTL_Buf1InfoUpdate/2
  Signal Conversion106/1 -> LM_OTL_Buf1InfoUpdate/19
  Signal Conversion105/1 -> LM_OTL_Buf1InfoUpdate/18
  Signal Conversion103/1 -> LM_OTL_Buf1InfoUpdate/16
  Signal Conversion104/1 -> LM_OTL_Buf1InfoUpdate/17
  Signal Conversion102/1 -> LM_OTL_Buf1InfoUpdate/15
  Signal Conversion101/1 -> LM_OTL_Buf1InfoUpdate/14
  Signal Conversion100/1 -> LM_OTL_Buf1InfoUpdate/13
  Signal Conversion99/1 -> LM_OTL_Buf1InfoUpdate/12
  Signal Conversion98/1 -> LM_OTL_Buf1InfoUpdate/11
  Signal Conversion114/1 -> LM_OTL_Buf1InfoUpdate/8
  Signal Conversion115/1 -> LM_OTL_Buf1InfoUpdate/9
  Signal Conversion113/1 -> LM_OTL_Buf1InfoUpdate/7
  Signal Conversion112/1 -> LM_OTL_Buf1InfoUpdate/6
  Signal Conversion111/1 -> LM_OTL_Buf1InfoUpdate/5
  Signal Conversion110/1 -> LM_OTL_Buf1InfoUpdate/4
  Signal Conversion109/1 -> LM_OTL_Buf1InfoUpdate/3
  Signal Conversion108/1 -> LM_OTL_Buf1InfoUpdate/20
  Signal Conversion78/1 -> LM_OTL_Buf2InfoUpdate/11
  Signal Conversion89/1 -> LM_OTL_Buf2InfoUpdate/21
  Signal Conversion87/1 -> LM_OTL_Buf2InfoUpdate/20
  Signal Conversion86/1 -> LM_OTL_Buf2InfoUpdate/19
  Signal Conversion85/1 -> LM_OTL_Buf2InfoUpdate/18
  Signal Conversion84/1 -> LM_OTL_Buf2InfoUpdate/17
  Signal Conversion82/1 -> LM_OTL_Buf2InfoUpdate/15
  Signal Conversion83/1 -> LM_OTL_Buf2InfoUpdate/16
  Signal Conversion80/1 -> LM_OTL_Buf2InfoUpdate/13
  Signal Conversion81/1 -> LM_OTL_Buf2InfoUpdate/14
  Signal Conversion79/1 -> LM_OTL_Buf2InfoUpdate/12
  Signal Conversion91/1 -> LM_OTL_Buf2InfoUpdate/5
  Signal Conversion96/1 -> LM_OTL_Buf2InfoUpdate/10
  Signal Conversion94/1 -> LM_OTL_Buf2InfoUpdate/8
  Signal Conversion95/1 -> LM_OTL_Buf2InfoUpdate/9
  Signal Conversion93/1 -> LM_OTL_Buf2InfoUpdate/7
  Signal Conversion92/1 -> LM_OTL_Buf2InfoUpdate/6
  Bus Selector/1 -> Signal Conversion110/1  "<LM_OTLCurLeLaObj1RcdedFlg>"
  Bus Selector/2 -> Signal Conversion111/1  "<LM_OTLCurLeLaObj2RcdedFlg>"
  Bus Selector1/1 -> Signal Conversion112/1  "<LM_OTLCurLeLaObj1RcdFlg>"
  Bus Selector1/2 -> Signal Conversion113/1  "<LM_OTLCurLeLaObj2RcdFlg>"
  Bus Selector2/1 -> Signal Conversion114/1  "<LM_OTLCurLeLaObj1ID>"
  Bus Selector2/2 -> Signal Conversion115/1  "<LM_OTLCurLeLaObj2ID>"
  Bus Selector3/1 -> Signal Conversion97/1  "<LM_OTLCurLeLaObj1Dx>"
  Bus Selector3/2 -> Signal Conversion98/1  "<LM_OTLCurLeLaObj2Dx>"
  Bus Selector3/3 -> Signal Conversion99/1  "<LM_OTLCurLeLaObj1Dy>"
  Bus Selector3/4 -> Signal Conversion100/1  "<LM_OTLCurLeLaObj2Dy>"
  Bus Selector4/1 -> Signal Conversion101/1  "<LM_OTLBufL1PNum>"
  Bus Selector4/2 -> Signal Conversion102/1  "<LM_OTLBufL1SPPos>"
  Bus Selector4/3 -> Signal Conversion103/1  "<LM_OTLBufL1EPPos>"
  Bus Selector5/1 -> Signal Conversion104/1  "<LM_OTLCurLeLaObj1Index>"
  Bus Selector5/2 -> Signal Conversion105/1  "<LM_OTLCurLeLaObj2Index>"
  Bus Selector6/1 -> Signal Conversion106/1  "<LM_OTLBufL1LastTPValid>"
  Bus Selector6/2 -> Signal Conversion108/1  "<LM_OTLBufL1LastEPPos>"
  Bus Selector7/1 -> Signal Conversion107/1  "<LM_OTLBufL1DxVectK1Adju>"
  Bus Selector7/2 -> Signal Conversion109/1  "<LM_OTLBufL1DyVectK1Adju>"
  Constant/1 -> LM_OTL_Buf1InfoUpdate/1
  Constant1/1 -> LM_OTL_Buf2InfoUpdate/2
  Bus Selector15/2 -> Signal Conversion90/1  "<LM_OTLBufL2DyVectK1Adju>"
  Bus Selector15/1 -> Signal Conversion88/1  "<LM_OTLBufL2DxVectK1Adju>"
  Bus Selector14/2 -> Signal Conversion89/1  "<LM_OTLBufL2LastEPPos>"
  Bus Selector14/1 -> Signal Conversion87/1  "<LM_OTLBufL2LastTPValid>"
  Bus Selector13/2 -> Signal Conversion86/1  "<LM_OTLCurLeLaObj2Index>"
  Bus Selector13/1 -> Signal Conversion85/1  "<LM_OTLCurLeLaObj1Index>"
  Bus Selector12/3 -> Signal Conversion84/1  "<LM_OTLBufL2EPPos>"
  Bus Selector12/2 -> Signal Conversion83/1  "<LM_OTLBufL2SPPos>"
  Bus Selector12/1 -> Signal Conversion82/1  "<LM_OTLBufL2PNum>"
  Bus Selector11/4 -> Signal Conversion81/1  "<LM_OTLCurLeLaObj2Dy>"
  Bus Selector11/3 -> Signal Conversion80/1  "<LM_OTLCurLeLaObj1Dy>"
  Bus Selector11/2 -> Signal Conversion79/1  "<LM_OTLCurLeLaObj2Dx>"
  Bus Selector11/1 -> Signal Conversion78/1  "<LM_OTLCurLeLaObj1Dx>"
  Bus Selector10/2 -> Signal Conversion96/1  "<LM_OTLCurLeLaObj2ID>"
  Bus Selector10/1 -> Signal Conversion95/1  "<LM_OTLCurLeLaObj1ID>"
  Bus Selector9/2 -> Signal Conversion94/1  "<LM_OTLCurLeLaObj2RcdFlg>"
  Bus Selector9/1 -> Signal Conversion93/1  "<LM_OTLCurLeLaObj1RcdFlg>"
  Bus Selector8/2 -> Signal Conversion92/1  "<LM_OTLCurLeLaObj2RcdedFlg>"
  Bus Selector8/1 -> Signal Conversion91/1  "<LM_OTLCurLeLaObj1RcdedFlg>"
  Signal Conversion88/1 -> LM_OTL_Buf2InfoUpdate/3
  Signal Conversion90/1 -> LM_OTL_Buf2InfoUpdate/4
  Bus Selector22/1 -> Signal Conversion4/1  "<LM_OTLCurEgoLaObj1RcdedFlg>"
  Bus Selector22/2 -> Signal Conversion5/1  "<LM_OTLCurEgoLaObj2RcdedFlg>"
  Bus Selector23/1 -> Signal Conversion6/1  "<LM_OTLCurEgoLaObj1RcdFlg>"
  Bus Selector23/2 -> Signal Conversion7/1  "<LM_OTLCurEgoLaObj2RcdFlg>"
  Bus Selector16/1 -> Signal Conversion8/1  "<LM_OTLCurEgoLaObj1ID>"
  Bus Selector16/2 -> Signal Conversion9/1  "<LM_OTLCurEgoLaObj2ID>"
  Bus Selector17/1 -> Signal Conversion10/1  "<LM_OTLCurEgoLaObj1Dx>"
  Bus Selector17/2 -> Signal Conversion11/1  "<LM_OTLCurEgoLaObj2Dx>"
  Bus Selector17/3 -> Signal Conversion12/1  "<LM_OTLCurEgoLaObj1Dy>"
  Bus Selector17/4 -> Signal Conversion13/1  "<LM_OTLCurEgoLaObj2Dy>"
  Bus Selector18/1 -> Signal Conversion14/1  "<LM_OTLBufE1PNum>"
  Bus Selector18/2 -> Signal Conversion15/1  "<LM_OTLBufE1SPPos>"
  Bus Selector18/3 -> Signal Conversion16/1  "<LM_OTLBufE1EPPos>"
  Bus Selector19/1 -> Signal Conversion17/1  "<LM_OTLCurEgoLaObj1Index>"
  Bus Selector19/2 -> Signal Conversion18/1  "<LM_OTLCurEgoLaObj2Index>"
  Bus Selector20/1 -> Signal Conversion19/1  "<LM_OTLBufE1LastTPValid>"
  Bus Selector20/2 -> Signal Conversion20/1  "<LM_OTLBufE1LastEPPos>"
  Bus Selector21/1 -> Signal Conversion2/1  "<LM_OTLBufE1DxVectK1Adju>"
  Bus Selector21/2 -> Signal Conversion3/1  "<LM_OTLBufE1DyVectK1Adju>"
  Constant2/1 -> LM_OTL_Buf1InfoUpdate1/1
  Signal Conversion2/1 -> LM_OTL_Buf1InfoUpdate1/2
  Signal Conversion3/1 -> LM_OTL_Buf1InfoUpdate1/3
  Signal Conversion4/1 -> LM_OTL_Buf1InfoUpdate1/4
  Signal Conversion5/1 -> LM_OTL_Buf1InfoUpdate1/5
  Signal Conversion6/1 -> LM_OTL_Buf1InfoUpdate1/6
  Signal Conversion7/1 -> LM_OTL_Buf1InfoUpdate1/7
  Signal Conversion8/1 -> LM_OTL_Buf1InfoUpdate1/8
  Signal Conversion9/1 -> LM_OTL_Buf1InfoUpdate1/9
  Signal Conversion10/1 -> LM_OTL_Buf1InfoUpdate1/10
  Signal Conversion11/1 -> LM_OTL_Buf1InfoUpdate1/11
  Signal Conversion12/1 -> LM_OTL_Buf1InfoUpdate1/12
  Signal Conversion13/1 -> LM_OTL_Buf1InfoUpdate1/13
  Signal Conversion15/1 -> LM_OTL_Buf1InfoUpdate1/15
  Signal Conversion14/1 -> LM_OTL_Buf1InfoUpdate1/14
  Signal Conversion16/1 -> LM_OTL_Buf1InfoUpdate1/16
  Signal Conversion17/1 -> LM_OTL_Buf1InfoUpdate1/17
  Signal Conversion18/1 -> LM_OTL_Buf1InfoUpdate1/18
  Signal Conversion19/1 -> LM_OTL_Buf1InfoUpdate1/19
  Signal Conversion20/1 -> LM_OTL_Buf1InfoUpdate1/20
  Signal Conversion32/1 -> LM_OTL_Buf2InfoUpdate1/21
  Signal Conversion30/1 -> LM_OTL_Buf2InfoUpdate1/20
  Signal Conversion29/1 -> LM_OTL_Buf2InfoUpdate1/19
  Signal Conversion28/1 -> LM_OTL_Buf2InfoUpdate1/18
  Signal Conversion27/1 -> LM_OTL_Buf2InfoUpdate1/17
  Signal Conversion25/1 -> LM_OTL_Buf2InfoUpdate1/15
  Signal Conversion26/1 -> LM_OTL_Buf2InfoUpdate1/16
  Signal Conversion24/1 -> LM_OTL_Buf2InfoUpdate1/14
  Signal Conversion23/1 -> LM_OTL_Buf2InfoUpdate1/13
  Signal Conversion22/1 -> LM_OTL_Buf2InfoUpdate1/12
  Signal Conversion21/1 -> LM_OTL_Buf2InfoUpdate1/11
  Signal Conversion39/1 -> LM_OTL_Buf2InfoUpdate1/10
  Signal Conversion38/1 -> LM_OTL_Buf2InfoUpdate1/9
  Signal Conversion37/1 -> LM_OTL_Buf2InfoUpdate1/8
  Signal Conversion36/1 -> LM_OTL_Buf2InfoUpdate1/7
  Signal Conversion35/1 -> LM_OTL_Buf2InfoUpdate1/6
  Signal Conversion34/1 -> LM_OTL_Buf2InfoUpdate1/5
  Signal Conversion33/1 -> LM_OTL_Buf2InfoUpdate1/4
  Signal Conversion31/1 -> LM_OTL_Buf2InfoUpdate1/3
  Constant3/1 -> LM_OTL_Buf2InfoUpdate1/2
  Bus Selector29/2 -> Signal Conversion33/1  "<LM_OTLBufE2DyVectK1Adju>"
  Bus Selector29/1 -> Signal Conversion31/1  "<LM_OTLBufE2DxVectK1Adju>"
  Bus Selector28/2 -> Signal Conversion32/1  "<LM_OTLBufE2LastEPPos>"
  Bus Selector28/1 -> Signal Conversion30/1  "<LM_OTLBufE2LastTPValid>"
  Bus Selector27/2 -> Signal Conversion29/1  "<LM_OTLCurEgoLaObj2Index>"
  Bus Selector27/1 -> Signal Conversion28/1  "<LM_OTLCurEgoLaObj1Index>"
  Bus Selector26/3 -> Signal Conversion27/1  "<LM_OTLBufE2EPPos>"
  Bus Selector26/2 -> Signal Conversion26/1  "<LM_OTLBufE2SPPos>"
  Bus Selector26/1 -> Signal Conversion25/1  "<LM_OTLBufE2PNum>"
  Bus Selector25/4 -> Signal Conversion24/1  "<LM_OTLCurEgoLaObj2Dy>"
  Bus Selector25/3 -> Signal Conversion23/1  "<LM_OTLCurEgoLaObj1Dy>"
  Bus Selector25/2 -> Signal Conversion22/1  "<LM_OTLCurEgoLaObj2Dx>"
  Bus Selector25/1 -> Signal Conversion21/1  "<LM_OTLCurEgoLaObj1Dx>"
  Bus Selector24/2 -> Signal Conversion39/1  "<LM_OTLCurEgoLaObj2ID>"
  Bus Selector24/1 -> Signal Conversion38/1  "<LM_OTLCurEgoLaObj1ID>"
  Bus Selector31/2 -> Signal Conversion37/1  "<LM_OTLCurEgoLaObj2RcdFlg>"
  Bus Selector31/1 -> Signal Conversion36/1  "<LM_OTLCurEgoLaObj1RcdFlg>"
  Bus Selector30/2 -> Signal Conversion35/1  "<LM_OTLCurEgoLaObj2RcdedFlg>"
  Bus Selector30/1 -> Signal Conversion34/1  "<LM_OTLCurEgoLaObj1RcdedFlg>"
  Bus Selector38/1 -> Signal Conversion53/1  "<LM_OTLCurRigLaObj1RcdedFlg>"
  Bus Selector38/2 -> Signal Conversion54/1  "<LM_OTLCurRigLaObj2RcdedFlg>"
  Bus Selector39/1 -> Signal Conversion55/1  "<LM_OTLCurRigLaObj1RcdFlg>"
  Bus Selector39/2 -> Signal Conversion56/1  "<LM_OTLCurRigLaObj2RcdFlg>"
  Bus Selector32/1 -> Signal Conversion57/1  "<LM_OTLCurRigLaObj1ID>"
  Bus Selector32/2 -> Signal Conversion58/1  "<LM_OTLCurRigLaObj2ID>"
  Bus Selector33/1 -> Signal Conversion40/1  "<LM_OTLCurRigLaObj1Dx>"
  Bus Selector33/2 -> Signal Conversion41/1  "<LM_OTLCurRigLaObj2Dx>"
  Bus Selector33/3 -> Signal Conversion42/1  "<LM_OTLCurRigLaObj1Dy>"
  Bus Selector33/4 -> Signal Conversion43/1  "<LM_OTLCurRigLaObj2Dy>"
  Bus Selector34/1 -> Signal Conversion44/1  "<LM_OTLBufR1PNum>"
  Bus Selector34/2 -> Signal Conversion45/1  "<LM_OTLBufR1SPPos>"
  Bus Selector34/3 -> Signal Conversion46/1  "<LM_OTLBufR1EPPos>"
  Bus Selector35/1 -> Signal Conversion47/1  "<LM_OTLCurRigLaObj1Index>"
  Bus Selector35/2 -> Signal Conversion48/1  "<LM_OTLCurRigLaObj2Index>"
  Bus Selector36/1 -> Signal Conversion49/1  "<LM_OTLBufR1LastTPValid>"
  Bus Selector36/2 -> Signal Conversion51/1  "<LM_OTLBufR1LastEPPos>"
  Bus Selector37/1 -> Signal Conversion50/1  "<LM_OTLBufR1DxVectK1Adju>"
  Bus Selector37/2 -> Signal Conversion52/1  "<LM_OTLBufR1DyVectK1Adju>"
  Constant4/1 -> LM_OTL_Buf1InfoUpdate2/1
  Signal Conversion50/1 -> LM_OTL_Buf1InfoUpdate2/2
  Signal Conversion52/1 -> LM_OTL_Buf1InfoUpdate2/3
  Signal Conversion53/1 -> LM_OTL_Buf1InfoUpdate2/4
  Signal Conversion54/1 -> LM_OTL_Buf1InfoUpdate2/5
  Signal Conversion55/1 -> LM_OTL_Buf1InfoUpdate2/6
  Signal Conversion56/1 -> LM_OTL_Buf1InfoUpdate2/7
  Signal Conversion57/1 -> LM_OTL_Buf1InfoUpdate2/8
  Signal Conversion58/1 -> LM_OTL_Buf1InfoUpdate2/9
  Signal Conversion40/1 -> LM_OTL_Buf1InfoUpdate2/10
  Signal Conversion41/1 -> LM_OTL_Buf1InfoUpdate2/11
  Signal Conversion42/1 -> LM_OTL_Buf1InfoUpdate2/12
  Signal Conversion43/1 -> LM_OTL_Buf1InfoUpdate2/13
  Signal Conversion45/1 -> LM_OTL_Buf1InfoUpdate2/15
  Signal Conversion44/1 -> LM_OTL_Buf1InfoUpdate2/14
  Signal Conversion46/1 -> LM_OTL_Buf1InfoUpdate2/16
  Signal Conversion47/1 -> LM_OTL_Buf1InfoUpdate2/17
  Signal Conversion48/1 -> LM_OTL_Buf1InfoUpdate2/18
  Signal Conversion49/1 -> LM_OTL_Buf1InfoUpdate2/19
  Signal Conversion51/1 -> LM_OTL_Buf1InfoUpdate2/20
  Signal Conversion70/1 -> LM_OTL_Buf2InfoUpdate2/21
  Signal Conversion68/1 -> LM_OTL_Buf2InfoUpdate2/20
  Signal Conversion67/1 -> LM_OTL_Buf2InfoUpdate2/19
  Signal Conversion66/1 -> LM_OTL_Buf2InfoUpdate2/18
  Signal Conversion65/1 -> LM_OTL_Buf2InfoUpdate2/17
  Signal Conversion63/1 -> LM_OTL_Buf2InfoUpdate2/15
  Signal Conversion64/1 -> LM_OTL_Buf2InfoUpdate2/16
  Signal Conversion62/1 -> LM_OTL_Buf2InfoUpdate2/14
  Signal Conversion61/1 -> LM_OTL_Buf2InfoUpdate2/13
  Signal Conversion60/1 -> LM_OTL_Buf2InfoUpdate2/12
  Signal Conversion59/1 -> LM_OTL_Buf2InfoUpdate2/11
  Signal Conversion77/1 -> LM_OTL_Buf2InfoUpdate2/10
  Signal Conversion76/1 -> LM_OTL_Buf2InfoUpdate2/9
  Signal Conversion75/1 -> LM_OTL_Buf2InfoUpdate2/8
  Signal Conversion74/1 -> LM_OTL_Buf2InfoUpdate2/7
  Signal Conversion73/1 -> LM_OTL_Buf2InfoUpdate2/6
  Signal Conversion72/1 -> LM_OTL_Buf2InfoUpdate2/5
  Signal Conversion71/1 -> LM_OTL_Buf2InfoUpdate2/4
  Signal Conversion69/1 -> LM_OTL_Buf2InfoUpdate2/3
  Constant5/1 -> LM_OTL_Buf2InfoUpdate2/2
  LM_OTLBufTPVectAdjuBus/1 -> Bus Selector21/1, Bus Selector45/1, Bus Selector37/1, Bus Selector29/1, Bus Selector15/1, Bus Selector7/1
  Bus Selector45/2 -> Signal Conversion71/1  "<LM_OTLBufR2DyVectK1Adju>"
  Bus Selector45/1 -> Signal Conversion69/1  "<LM_OTLBufR2DxVectK1Adju>"
  Bus Selector44/2 -> Signal Conversion70/1  "<LM_OTLBufR2LastEPPos>"
  Bus Selector44/1 -> Signal Conversion68/1  "<LM_OTLBufR2LastTPValid>"
  LM_OTLBufLastTPInfoBus/1 -> Bus Selector20/1, Bus Selector36/1, Subsystem/37(LM_OTLBufLastTPInfoBus), Bus Selector44/1, Bus Selector28/1, Bus Selector14/1, Bus Selector6/1
  LM_OTLInterestObjIndexBus/1 -> Bus Selector19/1, Bus Selector35/1, Bus Selector43/1, Bus Selector27/1, Bus Selector13/1, Bus Selector5/1
  Bus Selector43/2 -> Signal Conversion67/1  "<LM_OTLCurRigLaObj2Index>"
  Bus Selector43/1 -> Signal Conversion66/1  "<LM_OTLCurRigLaObj1Index>"
  Bus Selector42/3 -> Signal Conversion65/1  "<LM_OTLBufR2EPPos>"
  Bus Selector42/2 -> Signal Conversion64/1  "<LM_OTLBufR2SPPos>"
  Bus Selector42/1 -> Signal Conversion63/1  "<LM_OTLBufR2PNum>"
  LM_OTLBufTPInfoBusK1/1 -> Bus Selector18/1, Bus Selector34/1, Bus Selector42/1, Bus Selector26/1, Bus Selector12/1, Bus Selector4/1
  Bus Selector41/4 -> Signal Conversion62/1  "<LM_OTLCurRigLaObj2Dy>"
  Bus Selector41/3 -> Signal Conversion61/1  "<LM_OTLCurRigLaObj1Dy>"
  Bus Selector41/2 -> Signal Conversion60/1  "<LM_OTLCurRigLaObj2Dx>"
  Bus Selector41/1 -> Signal Conversion59/1  "<LM_OTLCurRigLaObj1Dx>"
  LM_OTLCurObjPositonBus/1 -> Bus Selector17/1, Bus Selector33/1, Bus Selector41/1, Bus Selector25/1, Bus Selector11/1, Bus Selector3/1
  Bus Selector40/2 -> Signal Conversion77/1  "<LM_OTLCurRigLaObj2ID>"
  Bus Selector40/1 -> Signal Conversion76/1  "<LM_OTLCurRigLaObj1ID>"
  LM_OTLCurObjIDBus/1 -> Bus Selector16/1, Bus Selector32/1, Bus Selector40/1, Bus Selector24/1, Bus Selector10/1, Bus Selector2/1
  Bus Selector47/2 -> Signal Conversion75/1  "<LM_OTLCurRigLaObj2RcdFlg>"
  Bus Selector47/1 -> Signal Conversion74/1  "<LM_OTLCurRigLaObj1RcdFlg>"
  LM_OTLCurObjRcdFlgBus/1 -> Bus Selector23/1, Bus Selector39/1, Bus Selector47/1, Bus Selector31/1, Bus Selector9/1, Bus Selector1/1
  Bus Selector46/2 -> Signal Conversion73/1  "<LM_OTLCurRigLaObj2RcdedFlg>"
  Bus Selector46/1 -> Signal Conversion72/1  "<LM_OTLCurRigLaObj1RcdedFlg>"
  LM_OTLObjRcdedFlg_Bus/1 -> Bus Selector22/1, Bus Selector38/1, Bus Selector46/1, Bus Selector30/1, Bus Selector8/1, Bus Selector/1
  LM_OTL_Buf1InfoUpdate/2 -> Subsystem/2(LM_OTLBufL1DyVect)
  LM_OTL_Buf1InfoUpdate/1 -> Subsystem/1(LM_OTLBufL1DxVect)
  LM_OTL_Buf1InfoUpdate/3 -> Subsystem/3(LM_OTLBufL1ObjID), LM_OTL_Buf2InfoUpdate/1
  LM_OTL_Buf1InfoUpdate/4 -> Subsystem/4(LM_OTLBufL1EPPos)
  LM_OTL_Buf1InfoUpdate/5 -> Subsystem/5(LM_OTLBufL1ObjTPNum)
  LM_OTL_Buf1InfoUpdate/6 -> Subsystem/6(LM_OTLBufL1SPPos)
  LM_OTL_Buf2InfoUpdate/1 -> Subsystem/7(LM_OTLBufL2DxVect)
  LM_OTL_Buf2InfoUpdate/2 -> Subsystem/8(LM_OTLBufL2DyVect)
  LM_OTL_Buf2InfoUpdate/3 -> Subsystem/9(LM_OTLBufL2ObjID)
  LM_OTL_Buf2InfoUpdate/4 -> Subsystem/10(LM_OTLBufL2EPPos)
  LM_OTL_Buf2InfoUpdate/5 -> Subsystem/11(LM_OTLBufL2ObjTPNum)
  LM_OTL_Buf2InfoUpdate/6 -> Subsystem/12(LM_OTLBufL2SPPos)
  LM_OTL_Buf1InfoUpdate1/1 -> Subsystem/13(LM_OTLBufE1DxVect)
  LM_OTL_Buf1InfoUpdate1/2 -> Subsystem/14(LM_OTLBufE1DyVect)
  LM_OTL_Buf1InfoUpdate1/3 -> Subsystem/15(LM_OTLBufE1ObjID), LM_OTL_Buf2InfoUpdate1/1
  LM_OTL_Buf1InfoUpdate1/4 -> Subsystem/16(LM_OTLBufE1EPPos)
  LM_OTL_Buf1InfoUpdate1/5 -> Subsystem/17(LM_OTLBufE1ObjTPNum)
  LM_OTL_Buf1InfoUpdate1/6 -> Subsystem/18(LM_OTLBufE1SPPos)
  LM_OTL_Buf2InfoUpdate1/1 -> Subsystem/19(LM_OTLBufE2DxVect)
  LM_OTL_Buf2InfoUpdate1/2 -> Subsystem/20(LM_OTLBufE2DyVect)
  LM_OTL_Buf2InfoUpdate1/3 -> Subsystem/21(LM_OTLBufE2ObjID)
  LM_OTL_Buf2InfoUpdate1/4 -> Subsystem/22(LM_OTLBufE2EPPos)
  LM_OTL_Buf2InfoUpdate1/5 -> Subsystem/23(LM_OTLBufE2ObjTPNum)
  LM_OTL_Buf2InfoUpdate1/6 -> Subsystem/24(LM_OTLBufLE2SPPos)
  LM_OTL_Buf1InfoUpdate2/1 -> Subsystem/25(LM_OTLBufR1DxVect)
  LM_OTL_Buf1InfoUpdate2/2 -> Subsystem/26(LM_OTLBufR1DyVect)
  LM_OTL_Buf1InfoUpdate2/3 -> Subsystem/27(LM_OTLBufR1ObjID), LM_OTL_Buf2InfoUpdate2/1
  LM_OTL_Buf1InfoUpdate2/4 -> Subsystem/28(LM_OTLBufR1EPPos)
  LM_OTL_Buf1InfoUpdate2/5 -> Subsystem/29(LM_OTLBufR1ObjTPNum)
  LM_OTL_Buf1InfoUpdate2/6 -> Subsystem/30(LM_OTLBufR1SPPos)
  LM_OTL_Buf2InfoUpdate2/1 -> Subsystem/31(LM_OTLBufR2DxVect)
  LM_OTL_Buf2InfoUpdate2/2 -> Subsystem/32(LM_OTLBufR2DyVect)
  LM_OTL_Buf2InfoUpdate2/3 -> Subsystem/33(LM_OTLBufR2ObjID)
  LM_OTL_Buf2InfoUpdate2/4 -> Subsystem/34(LM_OTLBufR2EPPos)
  LM_OTL_Buf2InfoUpdate2/5 -> Subsystem/35(LM_OTLBufR2ObjTPNum)
  LM_OTL_Buf2InfoUpdate2/6 -> Subsystem/36(LM_OTLBufR2SPPos)
  Subsystem/2(LM_OTLBufTPInfoBus) -> LM_OTLBufTPInfoBus/1
  Subsystem/1(LM_OTLBufTPVectBus) -> LM_OTLBufTPVectBus/1

== system PubIfDecisionLM_MDL/Subsystem2/LM_SigPrePro1/Subsystem1/LM_RFMLineInfoFilter ==
  RFM_LINE_L1 : Inport
  RFM_LINE_R1 : Inport  Port=2
  RFM_LINE_L2 : Inport  Port=3
  RFM_LINE_R2 : Inport  Port=4
  RFM_LINE_L3 : Inport  Port=5
  RFM_LINE_R3 : Inport  Port=6
  RFM_LINE_CL : Inport  Port=7
  RFM_LINE_LB : Inport  Port=8
  RFM_LINE_RB : Inport  Port=9
  Bus Creator : BusCreator  Inputs=10
  Bus Creator2 : BusCreator  Inputs=4
  Chart1 : Stateflow chart  AncestorBlock=LM_LIB/Chart2  TreatAsAtomicUnit=on
  Chart10 : Stateflow chart  Commented=on  TreatAsAtomicUnit=on
  Chart11 : Stateflow chart  Commented=on  TreatAsAtomicUnit=on
  Chart2 : Stateflow chart  AncestorBlock=LM_LIB/Chart2  TreatAsAtomicUnit=on
  Chart{3..9} (7 alike) : LM_LIB/Chart2  SystemSampleTime=-1  VariantActivationTime=update diagram  Latency=0  AutoFrameSizeCalculation=off
  Signal Conversion{2..19} (18 alike) : SignalConversion  OverrideOpt=off
  Unit Delay{1..9} (9 alike) : UnitDelay  SampleTime=-1  HasFrameUpgradeWarning=on
  LM_InputLineInfo : Outport
  wires:
  RFM_LINE_R1/1 -> Signal Conversion2/1, Bus Creator2/2  "RFM_LINE_R1"
  RFM_LINE_R2/1 -> Signal Conversion6/1, Bus Creator2/4  "RFM_LINE_R2"
  Bus Creator2/1 -> Bus Creator/1  "RFM_LINE"
  RFM_LINE_L1/1 -> Signal Conversion3/1, Bus Creator2/1  "RFM_LINE_L1"
  RFM_LINE_L2/1 -> Signal Conversion7/1, Bus Creator2/3  "RFM_LINE_L2"
  RFM_LINE_CL/1 -> Signal Conversion15/1
  RFM_LINE_R3/1 -> Signal Conversion10/1
  RFM_LINE_L3/1 -> Signal Conversion11/1
  RFM_LINE_RB/1 -> Signal Conversion18/1
  Signal Conversion19/1 -> Bus Creator/10  "LM_LINE_RB"
  Unit Delay9/1 -> Chart9/2
  Signal Conversion12/1 -> Bus Creator/6  "LM_LINE_L3"
  Signal Conversion6/1 -> Chart4/1  "RFM_LINE"
  Unit Delay3/1 -> Chart4/2
  Chart4/1 -> Signal Conversion9/1, Unit Delay3/1
  Unit Delay4/1 -> Chart3/2
  Unit Delay1/1 -> Chart1/2(LM_LINE_K1)
  Signal Conversion3/1 -> Chart2/1(RFM_LINE)  "RFM_LINE"
  Unit Delay5/1 -> Chart6/2
  Signal Conversion18/1 -> Chart9/1  "RFM_LINE"
  Signal Conversion10/1 -> Chart6/1  "RFM_LINE"
  Signal Conversion4/1 -> Bus Creator/2  "LM_LINE_L1"
  Signal Conversion16/1 -> Bus Creator/8  "LM_LINE_CL"
  Chart5/1 -> Unit Delay6/1, Signal Conversion12/1
  Signal Conversion13/1 -> Bus Creator/7  "LM_LINE_R3"
  Unit Delay8/1 -> Chart7/2
  Chart7/1 -> Unit Delay8/1, Signal Conversion16/1
  Chart3/1 -> Signal Conversion8/1, Unit Delay4/1
  Unit Delay7/1 -> Chart8/2
  Signal Conversion11/1 -> Chart5/1  "RFM_LINE"
  Signal Conversion15/1 -> Chart7/1  "RFM_LINE"
  Signal Conversion8/1 -> Bus Creator/4  "LM_LINE_L2"
  Chart9/1 -> Signal Conversion19/1, Unit Delay9/1
  Signal Conversion5/1 -> Bus Creator/3  "LM_LINE_R1"
  Signal Conversion2/1 -> Chart1/1(RFM_LINE)  "RFM_LINE"
  Signal Conversion17/1 -> Bus Creator/9  "LM_LINE_LB"
  Chart1/1(LM_LINE_Filt) -> Signal Conversion5/1, Unit Delay1/1
  Signal Conversion14/1 -> Chart8/1  "RFM_LINE"
  Chart6/1 -> Unit Delay5/1, Signal Conversion13/1
  RFM_LINE_LB/1 -> Signal Conversion14/1
  Chart2/1(LM_LINE_Filt) -> Signal Conversion4/1, Unit Delay2/1
  Unit Delay2/1 -> Chart2/2(LM_LINE_K1)
  Chart8/1 -> Unit Delay7/1, Signal Conversion17/1
  Unit Delay6/1 -> Chart5/2
  Signal Conversion7/1 -> Chart3/1  "RFM_LINE"
  Bus Creator/1 -> LM_InputLineInfo/1  "LM_InputLineInfo"
  Signal Conversion9/1 -> Bus Creator/5  "LM_LINE_R2"
